simulink model "lev4coilsSubs"  (R2021b)
settings: Solver=ode3  StartTime=0.0  StopTime=30  FixedStep=1e-3  RelTol=1e-3
values from neighbouring files (symbols this model uses):
  g = s(1:n,n+1:n+nb)    [MagLev.m]    (also in MagLev4coils.m = 9.8)
  K1 = m*g/(2*b)    (= 5.40205233157e-05)    [MagLev4coils.m]
  K2 = K1    (= 5.40205233157e-05)    [MagLev4coils.m]
  K3 = K1    (= 5.40205233157e-05)    [MagLev4coils.m]
  K4 = K2    (= 5.40205233157e-05)    [MagLev4coils.m]
  l = 0.0567/2    (= 0.02835)    [MagLev4coils.m]
  L1 = L    (= 0.00388)    [MagLev4coils.m]
  L2 = L    (= 0.00388)    [MagLev4coils.m]
  m = 0.03    [MagLev.m]    (also in MagLev4coils.m = 0.01)
  R1 = R    (= 4)    [MagLev4coils.m]
  R2 = R    (= 4)    [MagLev4coils.m]
settings Model: Creator=macbook_pro  LastModifiedBy=ik76

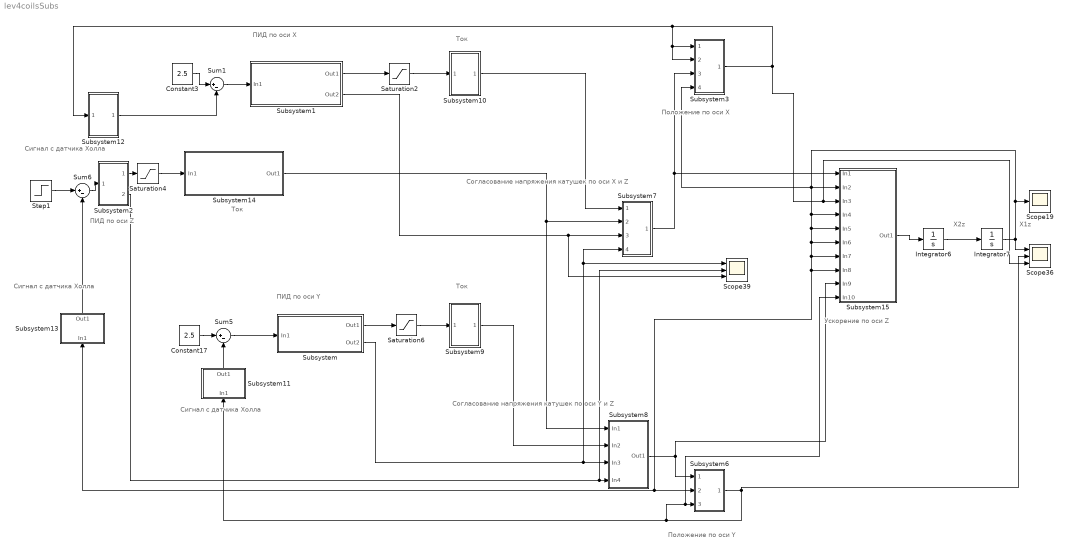
== system lev4coilsSubs ==
  note: Положение по оси X
  note: Согласование напряжения катушек по оси X и Z
  note: Положение по оси Y
  note: Ускорение по оси Z
  note: ПИД по оси Z
  note: Ток
  note: Сигнал с датчика Холла
  note: Согласование напряжения катушек по оси Y и Z
  note: ПИД по оси X
  note: ПИД по оси Y
  note: Сигнал с датчика Холла
  note: Сигнал с датчика Холла
  note: Ток
  note: Ток
  note: X2z
  note: X1z
  Constant17 : Constant  Value=2.5
  Constant3 : Constant  Value=2.5
  Integrator6 : Integrator
  Integrator7 : Integrator  InitialCondition=-0.03
  Saturation2 : Saturate  UpperLimit=5  LowerLimit=-5
  Saturation4 : Saturate  UpperLimit=5  LowerLimit=-5
  Saturation6 : Saturate  UpperLimit=5  LowerLimit=-5
  Scope19 : Scope
  Scope36 : Scope  NumInputPorts=3
  Scope39 : Scope  NumInputPorts=3
  Step1 : Step  Time=0  After=3.5  SampleTime=0
  Subsystem : Subsystem
  Subsystem1 : Subsystem
  Subsystem10 : Subsystem
  Subsystem11 : Subsystem
  Subsystem12 : Subsystem
  Subsystem13 : Subsystem
  Subsystem14 : Subsystem
  Subsystem15 : Subsystem
  Subsystem2 : Subsystem
  Subsystem3 : Subsystem
  Subsystem6 : Subsystem
  Subsystem7 : Subsystem
  Subsystem8 : Subsystem
  Subsystem9 : Subsystem
  Sum1 : Sum  Inputs=|+-
  Sum5 : Sum  Inputs=|+-
  Sum6 : Sum  Inputs=|+-
  wires:
  Integrator6/1 -> Integrator7/1
  Step1/1 -> Sum6/1
  Constant3/1 -> Sum1/1
  Integrator7/1 -> Scope19/1, Subsystem15/4(In4), Subsystem15/5(In5), Subsystem15/6(In6), Subsystem15/7(In7), Subsystem15/8(In8), Subsystem13/1(In1), Subsystem6/2(In2), Subsystem3/4(In4), Subsystem15/2(In2), Scope36/1
  Constant17/1 -> Sum5/1
  Subsystem/2(Out2) -> Scope39/1, Subsystem7/4(In4), Subsystem8/3(In3)
  Sum5/1 -> Subsystem/1(In1)
  Subsystem/1(Out1) -> Saturation6/1
  Subsystem1/2(Out2) -> Scope39/3, Subsystem7/3(In3)
  Sum1/1 -> Subsystem1/1(In1)
  Subsystem1/1(Out1) -> Saturation2/1
  Subsystem2/2(Out2) -> Scope39/2, Subsystem8/4(In4)
  Sum6/1 -> Subsystem2/1(In1)
  Subsystem2/1(Out1) -> Saturation4/1
  Subsystem3/1(Out1) -> Subsystem12/1(In1), Subsystem3/2(In2), Subsystem3/1(In1), Scope36/3, Subsystem15/3(In3)
  Subsystem6/1(Out1) -> Scope36/2, Subsystem6/3(In3), Subsystem15/10(In10), Subsystem11/1(In1)
  Subsystem7/1(Out1) -> Subsystem3/3(In3), Subsystem15/1(In1)
  Subsystem8/1(Out1) -> Subsystem15/9(In9), Subsystem6/1(In1)
  Saturation6/1 -> Subsystem9/1(In1)
  Subsystem9/1(Out1) -> Subsystem8/2(In2)
  Saturation2/1 -> Subsystem10/1(In1)
  Subsystem10/1(Out1) -> Subsystem7/1(In1)
  Subsystem11/1(Out1) -> Sum5/2
  Subsystem12/1(Out1) -> Sum1/2
  Subsystem13/1(Out1) -> Sum6/2
  Subsystem14/1(Out1) -> Subsystem7/2(In2), Subsystem8/1(In1)
  Saturation4/1 -> Subsystem14/1(In1)
  Subsystem15/1(Out1) -> Integrator6/1

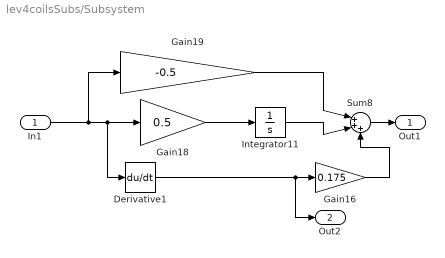
== system lev4coilsSubs/Subsystem ==
  In1 : Inport
  Derivative1 : Derivative
  Gain16 : Gain  Gain=0.175
  Gain18 : Gain  Gain=0.5
  Gain19 : Gain  Gain=-0.5
  Integrator11 : Integrator
  Sum8 : Sum  Inputs=|+++
  Out1 : Outport
  Out2 : Outport  Port=2
  wires:
  Sum8/1 -> Out1/1
  Gain19/1 -> Sum8/1
  In1/1 -> Gain19/1, Derivative1/1, Gain18/1
  Integrator11/1 -> Sum8/2
  Gain18/1 -> Integrator11/1
  Gain16/1 -> Sum8/3
  Derivative1/1 -> Gain16/1, Out2/1

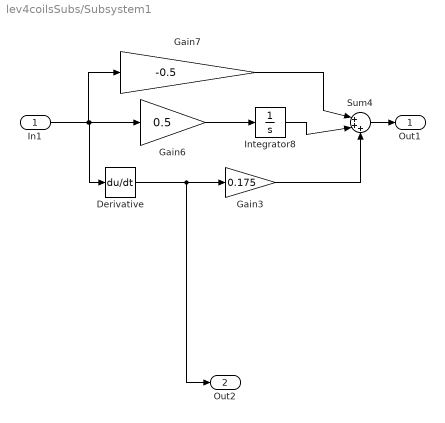
== system lev4coilsSubs/Subsystem1 ==
  In1 : Inport
  Derivative : Derivative
  Gain3 : Gain  Gain=0.175
  Gain6 : Gain  Gain=0.5
  Gain7 : Gain  Gain=-0.5
  Integrator8 : Integrator
  Sum4 : Sum  Inputs=|+++
  Out1 : Outport
  Out2 : Outport  Port=2
  wires:
  Derivative/1 -> Out2/1, Gain3/1
  Gain7/1 -> Sum4/1
  Gain3/1 -> Sum4/3
  In1/1 -> Gain7/1, Gain6/1, Derivative/1
  Sum4/1 -> Out1/1
  Gain6/1 -> Integrator8/1
  Integrator8/1 -> Sum4/2

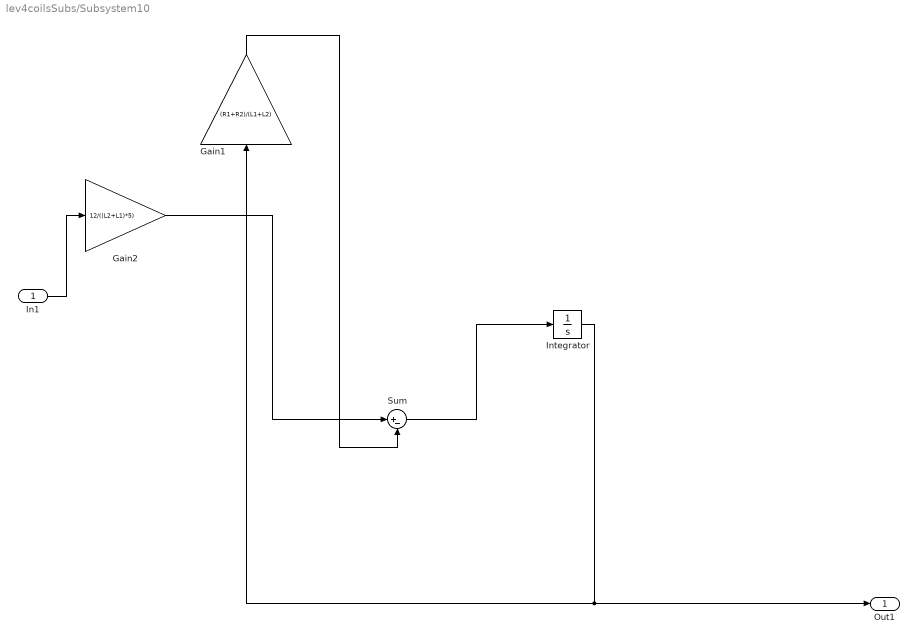
== system lev4coilsSubs/Subsystem10 ==
  In1 : Inport
  Gain1 : Gain  Gain=(R1+R2)/(L1+L2)
  Gain2 : Gain  Gain=12/((L2+L1)*5)
  Integrator : Integrator
  Sum : Sum  Inputs=|+-
  Out1 : Outport
  wires:
  Gain1/1 -> Sum/2
  In1/1 -> Gain2/1
  Gain2/1 -> Sum/1
  Sum/1 -> Integrator/1
  Integrator/1 -> Out1/1, Gain1/1

== system lev4coilsSubs/Subsystem11 ==
  In1 : Inport
  Constant22 : Constant  Value=2.5
  Gain17 : Gain  Gain=5/(l*2)
  Saturation3 : Saturate  UpperLimit=5  LowerLimit=0
  Subtract16 : Sum
  Out1 : Outport
  wires:
  Subtract16/1 -> Saturation3/1
  Gain17/1 -> Subtract16/2
  In1/1 -> Gain17/1
  Constant22/1 -> Subtract16/1
  Saturation3/1 -> Out1/1

== system lev4coilsSubs/Subsystem12 ==
  In1 : Inport
  Constant35 : Constant  Value=2.5
  Gain4 : Gain  Gain=5/(l*2)
  Saturation1 : Saturate  UpperLimit=5  LowerLimit=0
  Subtract27 : Sum
  Out1 : Outport
  wires:
  Constant35/1 -> Subtract27/1
  Subtract27/1 -> Saturation1/1
  Gain4/1 -> Subtract27/2
  In1/1 -> Gain4/1
  Saturation1/1 -> Out1/1

== system lev4coilsSubs/Subsystem13 ==
  In1 : Inport
  Abs10 : Abs
  Gain14 : Gain  Gain=(5/0.04)
  Saturation5 : Saturate  UpperLimit=0  LowerLimit=-5
  Out1 : Outport
  wires:
  Gain14/1 -> Saturation5/1
  Saturation5/1 -> Abs10/1
  In1/1 -> Gain14/1
  Abs10/1 -> Out1/1

== system lev4coilsSubs/Subsystem14 ==
  In1 : Inport
  Gain8 : Gain  Gain=(R1+R2)/(L1+L2)
  Gain9 : Gain  Gain=12/((L2+L1)*5)
  Integrator1 : Integrator
  Sum2 : Sum  Inputs=|+-
  Out1 : Outport
  wires:
  Gain9/1 -> Sum2/1
  Integrator1/1 -> Out1/1, Gain8/1
  In1/1 -> Gain9/1
  Gain8/1 -> Sum2/2
  Sum2/1 -> Integrator1/1

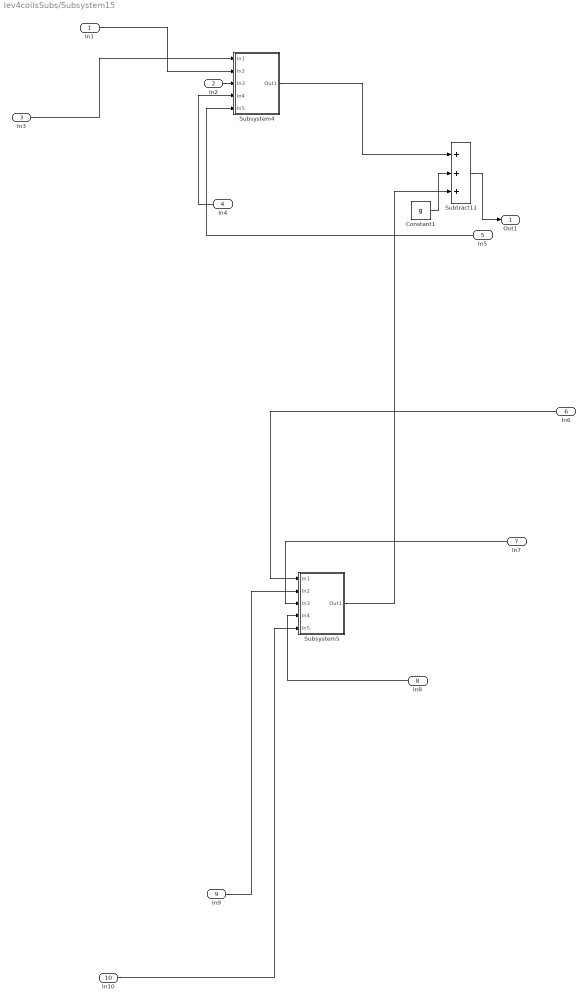
== system lev4coilsSubs/Subsystem15 ==
  In1 : Inport
  In2 : Inport  Port=2
  In3 : Inport  Port=3
  In4 : Inport  Port=4
  In5 : Inport  Port=5
  In6 : Inport  Port=6
  In7 : Inport  Port=7
  In8 : Inport  Port=8
  In9 : Inport  Port=9
  In10 : Inport  Port=10
  Constant1 : Constant  Value=g
  Subsystem4 : Subsystem
  Subsystem5 : Subsystem
  Subtract11 : Sum  Inputs=+++
  Out1 : Outport
  wires:
  In6/1 -> Subsystem5/1(In1)
  In9/1 -> Subsystem5/2(In2)
  Subsystem4/1(Out1) -> Subtract11/1
  Subsystem5/1(Out1) -> Subtract11/3
  In7/1 -> Subsystem5/3(In3)
  Constant1/1 -> Subtract11/2
  In8/1 -> Subsystem5/4(In4)
  Subtract11/1 -> Out1/1
  In10/1 -> Subsystem5/5(In5)
  In4/1 -> Subsystem4/4(In4)
  In5/1 -> Subsystem4/5(In5)
  In2/1 -> Subsystem4/3(In3)
  In1/1 -> Subsystem4/2(In2)
  In3/1 -> Subsystem4/1(In1)

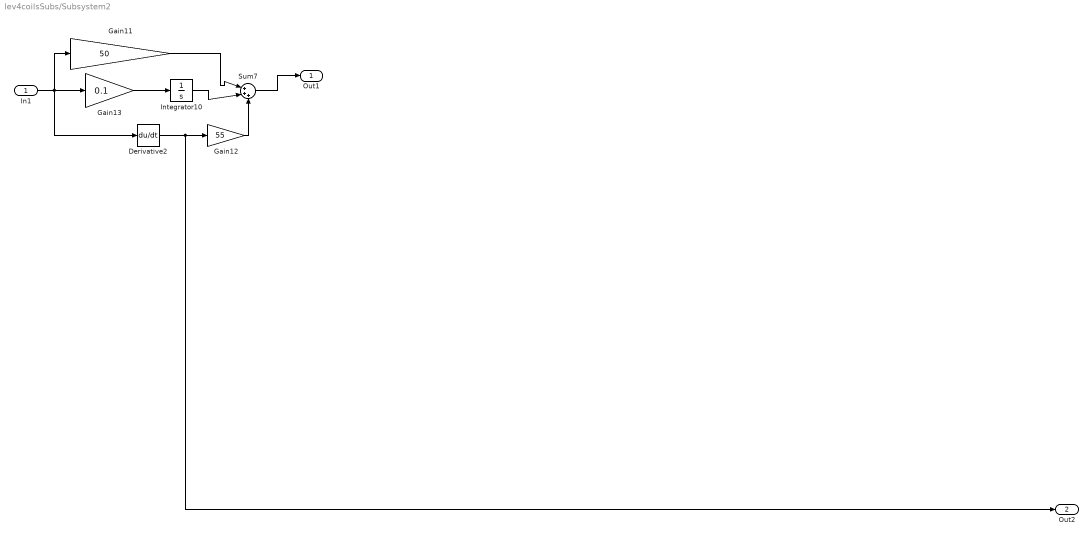
== system lev4coilsSubs/Subsystem2 ==
  In1 : Inport
  Derivative2 : Derivative
  Gain11 : Gain  Gain=50
  Gain12 : Gain  Gain=55
  Gain13 : Gain  Gain=0.1
  Integrator10 : Integrator
  Sum7 : Sum  Inputs=|+++
  Out1 : Outport
  Out2 : Outport  Port=2
  wires:
  Sum7/1 -> Out1/1
  Integrator10/1 -> Sum7/2
  In1/1 -> Derivative2/1, Gain13/1, Gain11/1
  Derivative2/1 -> Out2/1, Gain12/1
  Gain12/1 -> Sum7/3
  Gain11/1 -> Sum7/1
  Gain13/1 -> Integrator10/1

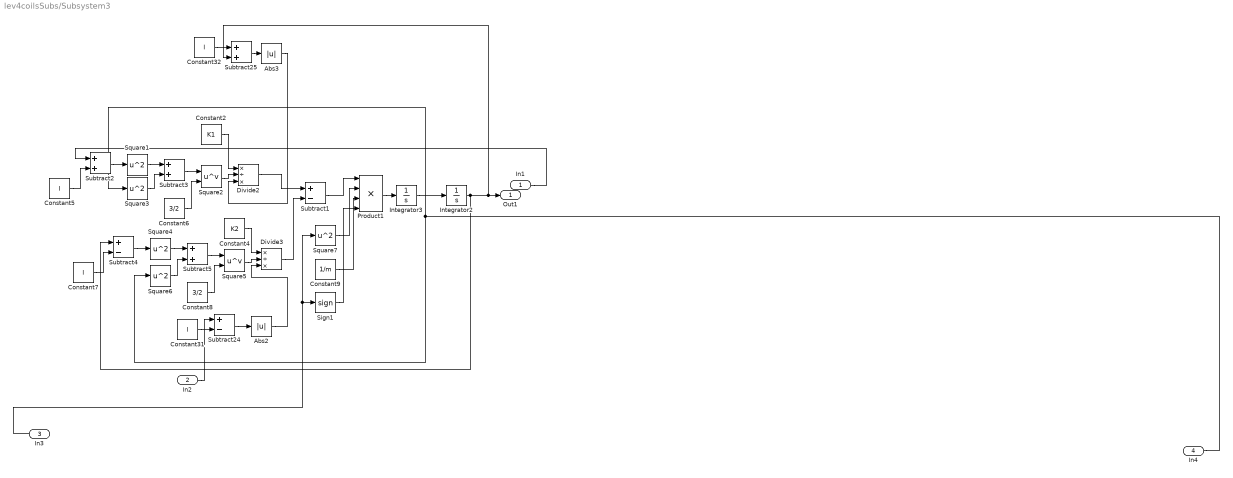
== system lev4coilsSubs/Subsystem3 ==
  In1 : Inport
  In2 : Inport  Port=2
  In3 : Inport  Port=3
  In4 : Inport  Port=4
  Abs2 : Abs
  Abs3 : Abs
  Constant2 : Constant  Value=K1
  Constant{5,7,31..32} (4 alike) : Constant  Value=l
  Constant4 : Constant  Value=K2
  Constant6 : Constant  Value=3/2
  Constant8 : Constant  Value=3/2
  Constant9 : Constant  Value=1/m
  Divide2 : Product  Inputs=*/*
  Divide3 : Product  Inputs=*/*
  Integrator2 : Integrator  InitialCondition=0.008
  Integrator3 : Integrator
  Product1 : Product  Inputs=4
  Sign1 : Signum
  Square{1,3..4,6..7} (5 alike) : Math  Operator=square  SaturateOnIntegerOverflow=on
  Square2 : Math  Operator=pow  SaturateOnIntegerOverflow=on
  Square5 : Math  Operator=pow  SaturateOnIntegerOverflow=on
  Subtract1 : Sum  Inputs=+-
  Subtract{2..3,5,25} (4 alike) : Sum
  Subtract24 : Sum  Inputs=+-
  Subtract4 : Sum  Inputs=+-
  Out1 : Outport
  wires:
  Square7/1 -> Product1/2
  In4/1 -> Square6/1, Square3/1
  Subtract5/1 -> Square5/1
  Product1/1 -> Integrator3/1
  In3/1 -> Square7/1, Sign1/1
  Constant6/1 -> Square2/2
  Constant8/1 -> Square5/2
  In2/1 -> Subtract24/1
  Divide3/1 -> Subtract1/2
  In1/1 -> Subtract2/1
  Sign1/1 -> Product1/4
  Square3/1 -> Subtract3/2
  Square4/1 -> Subtract5/1
  Constant7/1 -> Subtract4/2
  Constant32/1 -> Subtract25/1
  Subtract24/1 -> Abs2/1
  Constant4/1 -> Divide3/1
  Integrator2/1 -> Out1/1, Subtract25/2, Subtract4/1
  Square6/1 -> Subtract5/2
  Constant9/1 -> Product1/3
  Integrator3/1 -> Integrator2/1
  Divide2/1 -> Subtract1/1
  Abs3/1 -> Divide2/3
  Constant31/1 -> Subtract24/2
  Subtract3/1 -> Square2/1
  Constant5/1 -> Subtract2/2
  Subtract2/1 -> Square1/1
  Square1/1 -> Subtract3/1
  Subtract4/1 -> Square4/1
  Square5/1 -> Divide3/2
  Subtract1/1 -> Product1/1
  Subtract25/1 -> Abs3/1
  Square2/1 -> Divide2/2
  Abs2/1 -> Divide3/3
  Constant2/1 -> Divide2/1

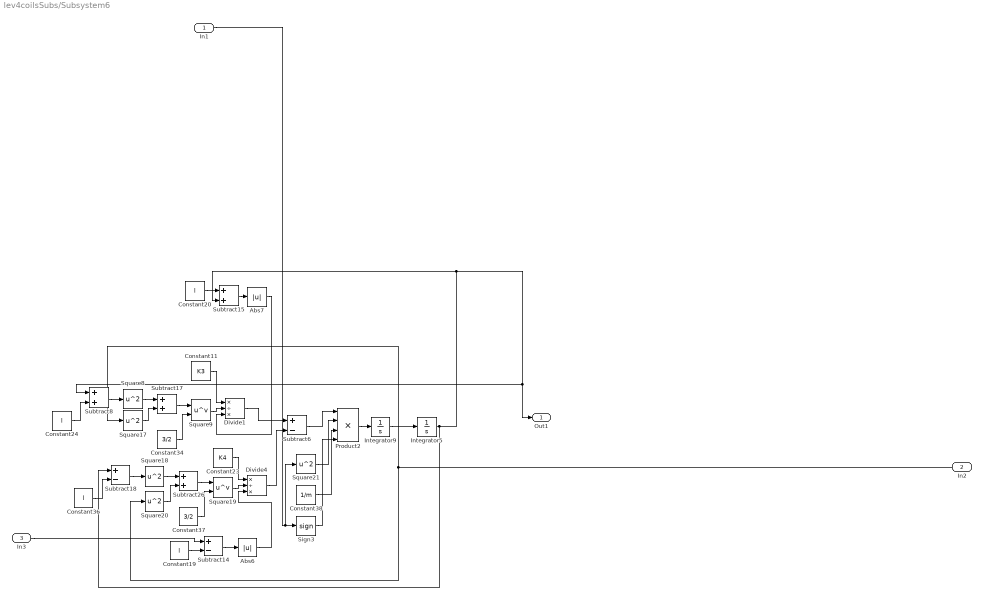
== system lev4coilsSubs/Subsystem6 ==
  In1 : Inport
  In2 : Inport  Port=2
  In3 : Inport  Port=3
  Abs6 : Abs
  Abs7 : Abs
  Constant11 : Constant  Value=K3
  Constant{19..20,24,36} (4 alike) : Constant  Value=l
  Constant23 : Constant  Value=K4
  Constant34 : Constant  Value=3/2
  Constant37 : Constant  Value=3/2
  Constant38 : Constant  Value=1/m
  Divide1 : Product  Inputs=*/*
  Divide4 : Product  Inputs=*/*
  Integrator5 : Integrator  InitialCondition=0.012
  Integrator9 : Integrator
  Product2 : Product  Inputs=4
  Sign3 : Signum
  Square{8,17..18,20..21} (5 alike) : Math  Operator=square  SaturateOnIntegerOverflow=on
  Square19 : Math  Operator=pow  SaturateOnIntegerOverflow=on
  Square9 : Math  Operator=pow  SaturateOnIntegerOverflow=on
  Subtract14 : Sum  Inputs=+-
  Subtract{8,15,17,26} (4 alike) : Sum
  Subtract18 : Sum  Inputs=+-
  Subtract6 : Sum  Inputs=+-
  Out1 : Outport
  wires:
  Constant34/1 -> Square9/2
  Subtract6/1 -> Product2/1
  Constant19/1 -> Subtract14/2
  Square8/1 -> Subtract17/1
  Square21/1 -> Product2/2
  Subtract26/1 -> Square19/1
  In2/1 -> Square20/1, Square17/1
  Constant11/1 -> Divide1/1
  Square20/1 -> Subtract26/2
  In3/1 -> Subtract14/1
  Divide1/1 -> Subtract6/1
  Subtract17/1 -> Square9/1
  Square18/1 -> Subtract26/1
  Square9/1 -> Divide1/2
  Constant20/1 -> Subtract15/1
  Constant36/1 -> Subtract18/2
  Subtract14/1 -> Abs6/1
  Constant38/1 -> Product2/3
  Integrator5/1 -> Out1/1, Subtract8/1, Subtract15/2, Subtract18/1
  Integrator9/1 -> Integrator5/1
  Abs6/1 -> Divide4/3
  Subtract8/1 -> Square8/1
  Product2/1 -> Integrator9/1
  Subtract18/1 -> Square18/1
  Divide4/1 -> Subtract6/2
  Square19/1 -> Divide4/2
  Square17/1 -> Subtract17/2
  Sign3/1 -> Product2/4
  Constant37/1 -> Square19/2
  Subtract15/1 -> Abs7/1
  In1/1 -> Square21/1, Sign3/1
  Abs7/1 -> Divide1/3
  Constant23/1 -> Divide4/1
  Constant24/1 -> Subtract8/2

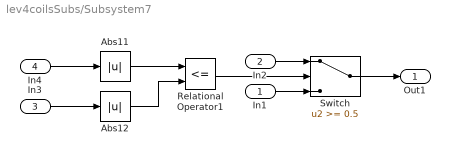
== system lev4coilsSubs/Subsystem7 ==
  In1 : Inport
  In2 : Inport  Port=2
  In3 : Inport  Port=3
  In4 : Inport  Port=4
  Abs11 : Abs
  Abs12 : Abs
  Relational Operator1 : RelationalOperator  Operator=<=  OutDataTypeStr=boolean  RndMeth=Simplest
  Switch : Switch  Threshold=0.5
  Out1 : Outport
  wires:
  In4/1 -> Abs11/1
  Abs11/1 -> Relational Operator1/1
  Relational Operator1/1 -> Switch/2
  Abs12/1 -> Relational Operator1/2
  In1/1 -> Switch/3
  In2/1 -> Switch/1
  In3/1 -> Abs12/1
  Switch/1 -> Out1/1

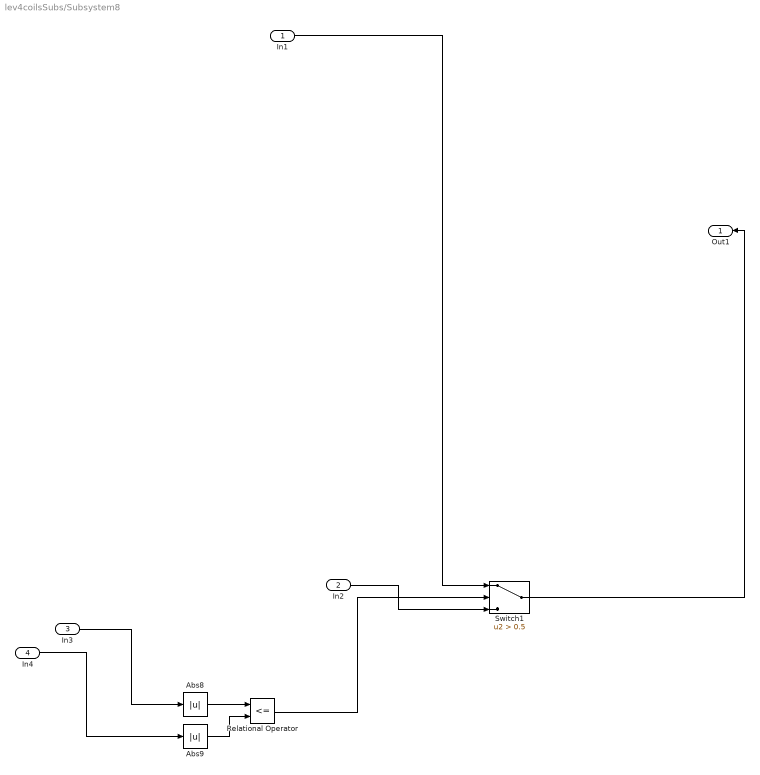
== system lev4coilsSubs/Subsystem8 ==
  In1 : Inport
  In2 : Inport  Port=2
  In3 : Inport  Port=3
  In4 : Inport  Port=4
  Abs8 : Abs
  Abs9 : Abs
  Relational Operator : RelationalOperator  Operator=<=  OutDataTypeStr=boolean  RndMeth=Simplest
  Switch1 : Switch  Criteria=u2 > Threshold  Threshold=0.5
  Out1 : Outport
  wires:
  Relational Operator/1 -> Switch1/2
  Abs8/1 -> Relational Operator/1
  Abs9/1 -> Relational Operator/2
  In1/1 -> Switch1/1
  In2/1 -> Switch1/3
  In4/1 -> Abs9/1
  Switch1/1 -> Out1/1
  In3/1 -> Abs8/1

== system lev4coilsSubs/Subsystem9 ==
  In1 : Inport
  Gain10 : Gain  Gain=(R1+R2)/(L1+L2)
  Gain15 : Gain  Gain=12/((L2+L1)*5)
  Integrator4 : Integrator
  Sum3 : Sum  Inputs=|+-
  Out1 : Outport
  wires:
  Sum3/1 -> Integrator4/1
  Integrator4/1 -> Out1/1, Gain10/1
  Gain15/1 -> Sum3/1
  Gain10/1 -> Sum3/2
  In1/1 -> Gain15/1

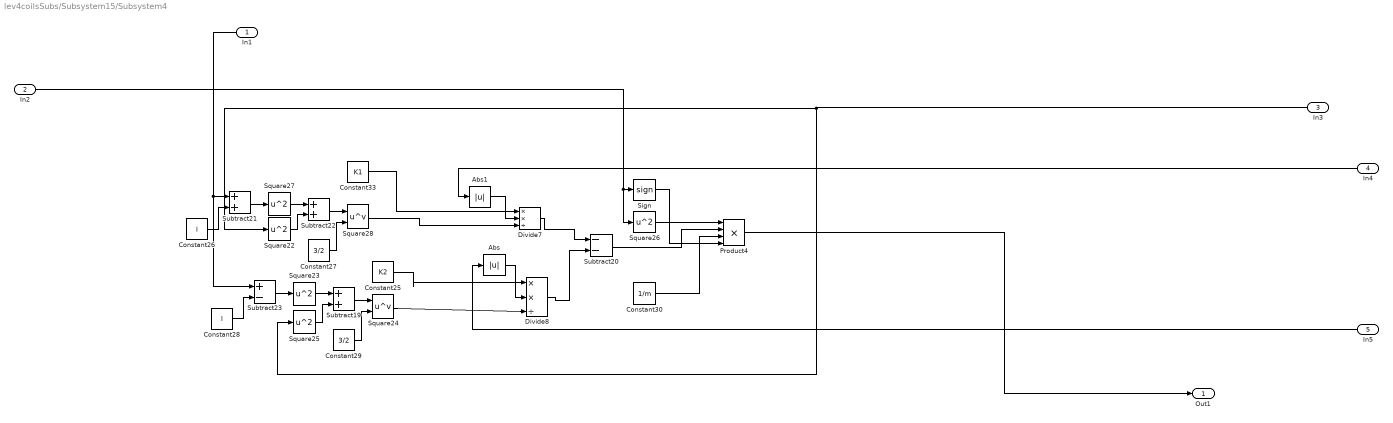
== system lev4coilsSubs/Subsystem15/Subsystem4 ==
  In1 : Inport
  In2 : Inport  Port=2
  In3 : Inport  Port=3
  In4 : Inport  Port=4
  In5 : Inport  Port=5
  Abs : Abs
  Abs1 : Abs
  Constant25 : Constant  Value=K2
  Constant26 : Constant  Value=l
  Constant27 : Constant  Value=3/2
  Constant28 : Constant  Value=l
  Constant29 : Constant  Value=3/2
  Constant30 : Constant  Value=1/m
  Constant33 : Constant  Value=K1
  Divide7 : Product  Inputs=**/
  Divide8 : Product  Inputs=**/
  Product4 : Product  Inputs=4
  Sign : Signum
  Square{22..23,25..27} (5 alike) : Math  Operator=square  SaturateOnIntegerOverflow=on
  Square24 : Math  Operator=pow  SaturateOnIntegerOverflow=on
  Square28 : Math  Operator=pow  SaturateOnIntegerOverflow=on
  Subtract19 : Sum
  Subtract20 : Sum  Inputs=--
  Subtract21 : Sum
  Subtract22 : Sum
  Subtract23 : Sum  Inputs=+-
  Out1 : Outport
  wires:
  In4/1 -> Abs1/1
  Sign/1 -> Product4/4
  Square22/1 -> Subtract22/2
  Square24/1 -> Divide8/3
  Subtract23/1 -> Square23/1
  Constant29/1 -> Square24/2
  Subtract21/1 -> Square27/1
  Subtract19/1 -> Square24/1
  In3/1 -> Square22/1, Square25/1
  Divide7/1 -> Subtract20/1
  Constant33/1 -> Divide7/1
  Square23/1 -> Subtract19/1
  In1/1 -> Subtract21/1, Subtract23/1
  In2/1 -> Square26/1, Sign/1
  Constant28/1 -> Subtract23/2
  Square25/1 -> Subtract19/2
  Subtract20/1 -> Product4/2
  Constant27/1 -> Square28/2
  Constant30/1 -> Product4/3
  Divide8/1 -> Subtract20/2
  Product4/1 -> Out1/1
  Constant26/1 -> Subtract21/2
  Square27/1 -> Subtract22/1
  Square28/1 -> Divide7/3
  Abs1/1 -> Divide7/2
  Square26/1 -> Product4/1
  Subtract22/1 -> Square28/1
  Abs/1 -> Divide8/2
  Constant25/1 -> Divide8/1
  In5/1 -> Abs/1

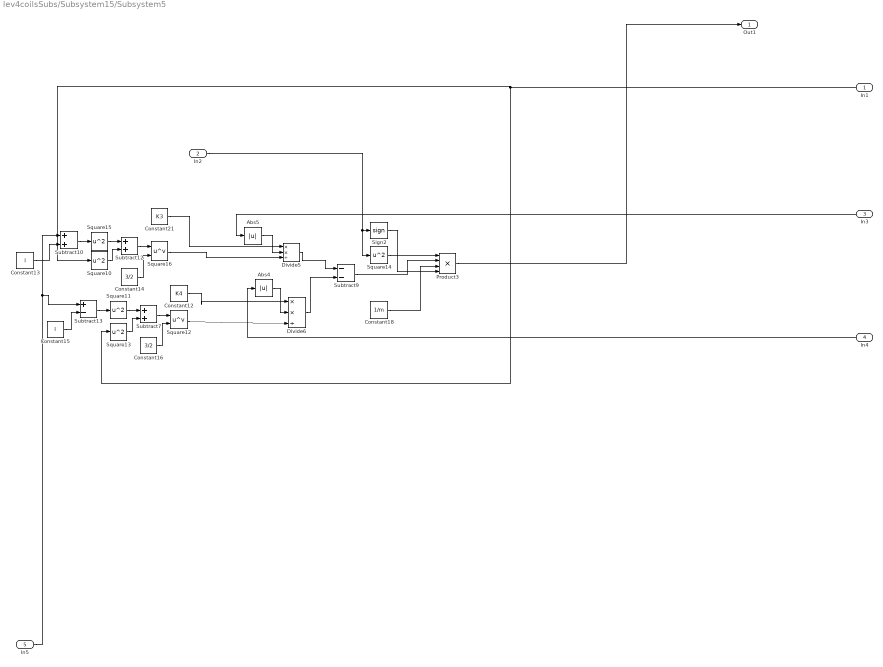
== system lev4coilsSubs/Subsystem15/Subsystem5 ==
  In1 : Inport
  In2 : Inport  Port=2
  In3 : Inport  Port=3
  In4 : Inport  Port=4
  In5 : Inport  Port=5
  Abs4 : Abs
  Abs5 : Abs
  Constant12 : Constant  Value=K4
  Constant13 : Constant  Value=l
  Constant14 : Constant  Value=3/2
  Constant15 : Constant  Value=l
  Constant16 : Constant  Value=3/2
  Constant18 : Constant  Value=1/m
  Constant21 : Constant  Value=K3
  Divide5 : Product  Inputs=**/
  Divide6 : Product  Inputs=**/
  Product3 : Product  Inputs=4
  Sign2 : Signum
  Square{10..11,13..15} (5 alike) : Math  Operator=square  SaturateOnIntegerOverflow=on
  Square12 : Math  Operator=pow  SaturateOnIntegerOverflow=on
  Square16 : Math  Operator=pow  SaturateOnIntegerOverflow=on
  Subtract10 : Sum
  Subtract12 : Sum
  Subtract13 : Sum  Inputs=+-
  Subtract7 : Sum
  Subtract9 : Sum  Inputs=--
  Out1 : Outport
  wires:
  Square15/1 -> Subtract12/1
  Constant12/1 -> Divide6/1
  Constant21/1 -> Divide5/1
  In5/1 -> Subtract10/1, Subtract13/1
  In1/1 -> Square10/1, Square13/1
  Subtract13/1 -> Square11/1
  Constant16/1 -> Square12/2
  Abs4/1 -> Divide6/2
  Square11/1 -> Subtract7/1
  Subtract12/1 -> Square16/1
  Square13/1 -> Subtract7/2
  Constant15/1 -> Subtract13/2
  Divide6/1 -> Subtract9/2
  Constant14/1 -> Square16/2
  Divide5/1 -> Subtract9/1
  Square10/1 -> Subtract12/2
  In2/1 -> Square14/1, Sign2/1
  Constant13/1 -> Subtract10/2
  Subtract9/1 -> Product3/2
  Subtract7/1 -> Square12/1
  Square12/1 -> Divide6/3
  Square16/1 -> Divide5/3
  Square14/1 -> Product3/1
  Subtract10/1 -> Square15/1
  Abs5/1 -> Divide5/2
  Sign2/1 -> Product3/4
  In4/1 -> Abs4/1
  Constant18/1 -> Product3/3
  In3/1 -> Abs5/1
  Product3/1 -> Out1/1
